simulink model "testerdolimiterow"  (R2022b)
settings: Solver=VariableStepAuto  StartTime=0.0  StopTime=10  RelTol=1e-3
values from neighbouring files (symbols this model uses):
  IPR = 0.99    [dane.m]    (also in tester23.m; wykresownik33.m; wykresownik35.m; wykresownik36.m)
  Ng_safe = 1.25    [dane.m]    (also in tester23.m; wykresownik33.m; wykresownik35.m; wykresownik36.m)
  No_perf = 1    [dane.m]    (also in tester23.m; wykresownik33.m; wykresownik35.m; wykresownik36.m)
  No_safe = 1.16    [dane.m]    (also in tester23.m; wykresownik33.m; wykresownik35.m; wykresownik36.m)
  Np = linspace(0.5,2,101)    [dane.m]    (also in tester23.m; untitled.m = 2303; wykresownik33.m; wykresownik35.m)
  Np_safe = 1.25    [dane.m]    (also in tester23.m; wykresownik33.m; wykresownik35.m; wykresownik36.m)
  P3tDIVP2t_perf = 1.0101    [dane.m]    (also in tester23.m = 1; wykresownik33.m = 1; wykresownik35.m = 1; wykresownik36.m = 1)
  Q = 1./Np    [dane.m]    (also in tester23.m; wykresownik33.m; wykresownik35.m; wykresownik36.m)
  Q_safe = 1.15    [dane.m]    (also in tester23.m; wykresownik33.m; wykresownik35.m; wykresownik36.m)
  T45_perf = 1    [dane.m]    (also in tester23.m; wykresownik33.m; wykresownik35.m; wykresownik36.m)
  T45_safe = 1.3    [dane.m]    (also in tester23.m; wykresownik33.m; wykresownik35.m; wykresownik36.m)
settings Model: Creator=48519  LastModifiedBy=48519
settings ModelReferenceCC: EnableRefExpFcnMdlSchedulingChecks=on

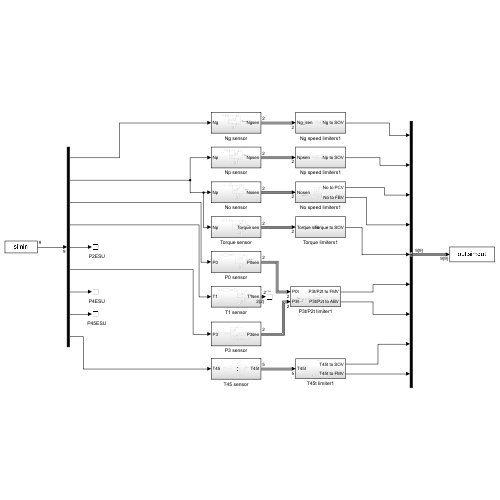
[thumbnail: Simulink's stored preview of the top-level diagram]
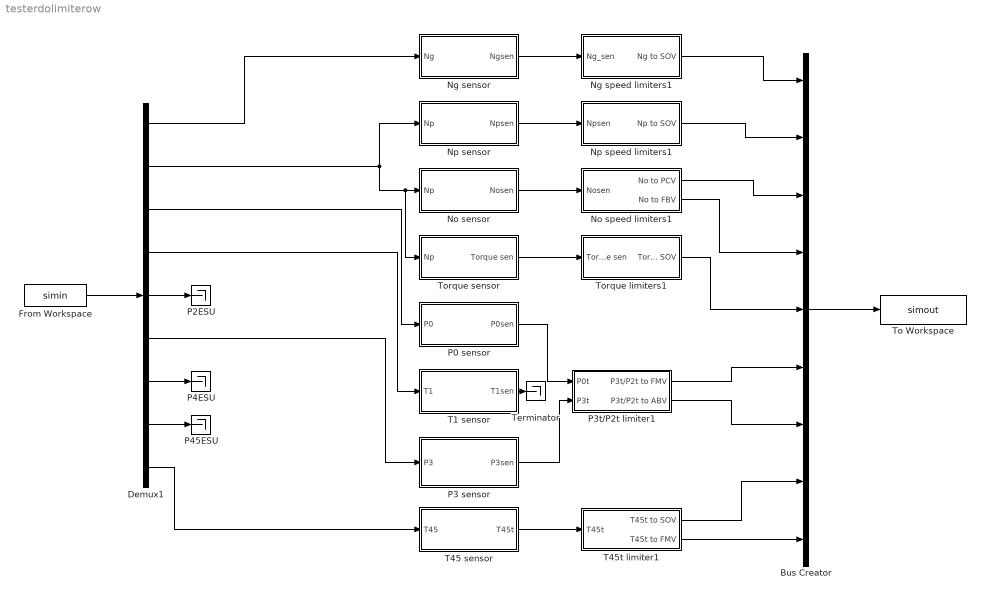
== system testerdolimiterow ==
  Bus Creator : BusCreator  Inputs=9
  Demux1 : Demux  Outputs=9
  From Workspace : FromWorkspace  VariableName=simin
  Ng sensor : Subsystem
  Ng speed limiters1 : Subsystem
  No sensor : Subsystem
  No speed limiters1 : Subsystem
  Np sensor : Subsystem
  Np speed limiters1 : Subsystem
  P0 sensor : Subsystem
  P2ESU : Terminator
  P3 sensor : Subsystem
  P3t/P2t limiter1 : Subsystem
  P45ESU : Terminator
  P4ESU : Terminator
  T1 sensor : Subsystem
  T45 sensor : Subsystem
  T45t limiter1 : Subsystem
  Terminator : Terminator
  To Workspace : ToWorkspace  VariableName=simout  SaveFormat=Timeseries  SampleTime=-1
  Torque limiters1 : Subsystem
  Torque sensor : Subsystem
  wires:
  Torque sensor/1(Torque sen) -> Torque limiters1/1(Torque sen)
  Ng sensor/1(Ngsen) -> Ng speed limiters1/1(Ng_sen)
  Demux1/2 -> Np sensor/1(Np), Torque sensor/1(Np), No sensor/1(Np)
  Demux1/1 -> Ng sensor/1(Ng)
  P3 sensor/1(P3sen) -> P3t/P2t limiter1/2(P3t)
  No sensor/1(Nosen) -> No speed limiters1/1(Nosen)
  P0 sensor/1(P0sen) -> P3t/P2t limiter1/1(P0t)
  From Workspace/1 -> Demux1/1
  Demux1/8 -> P45ESU/1
  Demux1/3 -> P0 sensor/1(P0)
  Demux1/6 -> P3 sensor/1(P3)
  Demux1/7 -> P4ESU/1
  Demux1/4 -> T1 sensor/1(T1)
  Demux1/5 -> P2ESU/1
  Demux1/9 -> T45 sensor/1(T45)
  Np sensor/1(Npsen) -> Np speed limiters1/1(Npsen)
  T45 sensor/1(T45t) -> T45t limiter1/1(T45t)
  T1 sensor/1(T1sen) -> Terminator/1
  P3t/P2t limiter1/2(P3t/P2t to ABV) -> Bus Creator/7
  Ng speed limiters1/1(Ng to SOV) -> Bus Creator/1
  T45t limiter1/1(T45t to SOV) -> Bus Creator/8
  Np speed limiters1/1(Np to SOV) -> Bus Creator/2
  No speed limiters1/1(No to PCV) -> Bus Creator/3
  Bus Creator/1 -> To Workspace/1
  No speed limiters1/2(No to FBV) -> Bus Creator/4
  P3t/P2t limiter1/1(P3t/P2t to FMV) -> Bus Creator/6
  T45t limiter1/2(T45t to FMV) -> Bus Creator/9
  Torque limiters1/1(Torque to SOV) -> Bus Creator/5

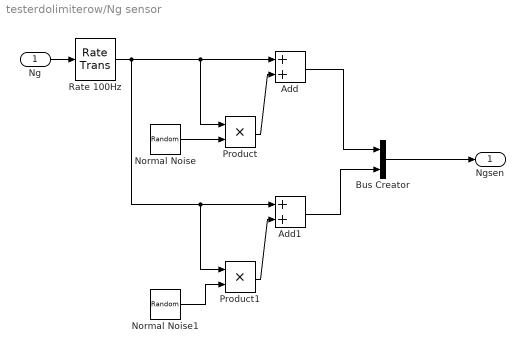
== system testerdolimiterow/Ng sensor ==
  Ng : Inport
  Add : Sum
  Add1 : Sum
  Bus Creator : BusCreator  Inputs=2
  Normal Noise : RandomNumber  Variance=((0.017)^2)*pi/2  Seed=10  SampleTime=0.01
  Normal Noise1 : RandomNumber  Variance=((0.017)^2)*pi/2  Seed=11  SampleTime=0.01
  Product : Product
  Product1 : Product
  Rate 100Hz : RateTransition  OutPortSampleTimeMultiple=2  OutPortSampleTime=0.01
  Ngsen : Outport
  wires:
  Product/1 -> Add/2
  Product1/1 -> Add1/2
  Normal Noise1/1 -> Product1/2
  Rate 100Hz/1 -> Add/1, Product/1, Add1/1, Product1/1
  Ng/1 -> Rate 100Hz/1
  Add1/1 -> Bus Creator/2
  Add/1 -> Bus Creator/1
  Bus Creator/1 -> Ngsen/1
  Normal Noise/1 -> Product/2

== system testerdolimiterow/Ng speed limiters1 ==
  Ng_sen : Inport
  Add : Sum
  Constant : Constant  Value=-1
  Constant1 : Constant
  Demux : Demux  Outputs=2
  Gain : Gain  Gain=0.5
  Safe switch : Subsystem
  Switch : Switch  Criteria=u2 > Threshold  Threshold=Ng_safe  SaturateOnIntegerOverflow=off  InputSameDT=off
  Ng to SOV : Outport
  wires:
  Constant/1 -> Switch/3
  Constant1/1 -> Switch/1
  Ng_sen/1 -> Demux/1
  Demux/1 -> Add/1
  Demux/2 -> Add/2
  Gain/1 -> Switch/2
  Add/1 -> Gain/1
  Switch/1 -> Safe switch/1(In1)
  Safe switch/1(Out1) -> Ng to SOV/1

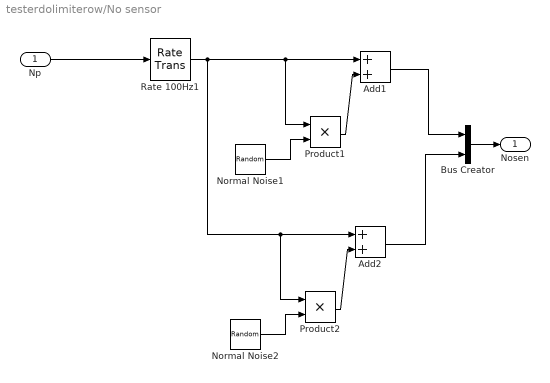
== system testerdolimiterow/No sensor ==
  Np : Inport
  Add1 : Sum
  Add2 : Sum
  Bus Creator : BusCreator  Inputs=2
  Normal Noise1 : RandomNumber  Variance=((0.017)^2)*pi/2  Seed=16  SampleTime=0.01
  Normal Noise2 : RandomNumber  Variance=((0.017)^2)*pi/2  Seed=18  SampleTime=0.01
  Product1 : Product
  Product2 : Product
  Rate 100Hz1 : RateTransition  OutPortSampleTimeMultiple=2  OutPortSampleTime=0.01
  Nosen : Outport
  wires:
  Np/1 -> Rate 100Hz1/1
  Normal Noise2/1 -> Product2/2
  Rate 100Hz1/1 -> Add2/1, Product2/1, Add1/1, Product1/1
  Add2/1 -> Bus Creator/2
  Add1/1 -> Bus Creator/1
  Bus Creator/1 -> Nosen/1
  Normal Noise1/1 -> Product1/2
  Product1/1 -> Add1/2
  Product2/1 -> Add2/2

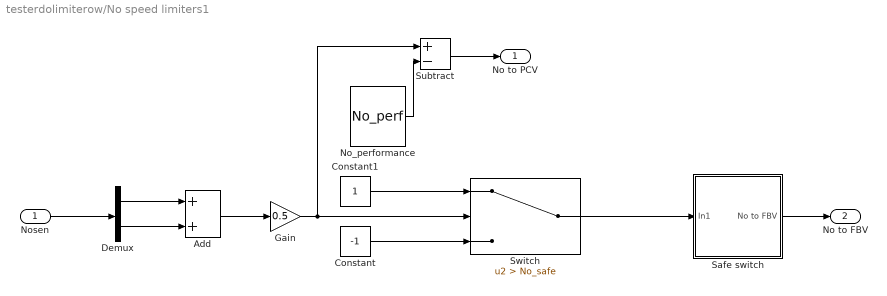
== system testerdolimiterow/No speed limiters1 ==
  Nosen : Inport
  Add : Sum
  Constant : Constant  Value=-1
  Constant1 : Constant
  Demux : Demux  Outputs=2
  Gain : Gain  Gain=0.5
  No_performance : Constant  Value=No_perf
  Safe switch : Subsystem
  Subtract : Sum  Inputs=+-
  Switch : Switch  Criteria=u2 > Threshold  Threshold=No_safe  SaturateOnIntegerOverflow=off  InputSameDT=off
  No to PCV : Outport
  No to FBV : Outport  Port=2
  wires:
  Add/1 -> Gain/1
  Nosen/1 -> Demux/1
  Demux/1 -> Add/1
  Demux/2 -> Add/2
  Constant/1 -> Switch/3
  Constant1/1 -> Switch/1
  Gain/1 -> Subtract/1, Switch/2
  No_performance/1 -> Subtract/2
  Subtract/1 -> No to PCV/1
  Switch/1 -> Safe switch/1(In1)
  Safe switch/1(No to FBV) -> No to FBV/1

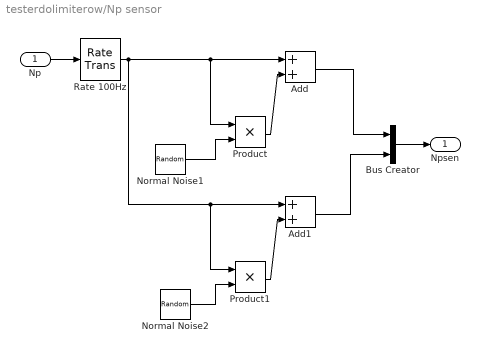
== system testerdolimiterow/Np sensor ==
  Np : Inport
  Add : Sum
  Add1 : Sum
  Bus Creator : BusCreator  Inputs=2
  Normal Noise1 : RandomNumber  Variance=((0.017)^2)*pi/2  Seed=13  SampleTime=0.01
  Normal Noise2 : RandomNumber  Variance=((0.017)^2)*pi/2  Seed=14  SampleTime=0.01
  Product : Product
  Product1 : Product
  Rate 100Hz : RateTransition  OutPortSampleTimeMultiple=2  OutPortSampleTime=0.01
  Npsen : Outport
  wires:
  Normal Noise1/1 -> Product/2
  Product/1 -> Add/2
  Np/1 -> Rate 100Hz/1
  Normal Noise2/1 -> Product1/2
  Product1/1 -> Add1/2
  Rate 100Hz/1 -> Add/1, Product/1, Add1/1, Product1/1
  Add1/1 -> Bus Creator/2
  Add/1 -> Bus Creator/1
  Bus Creator/1 -> Npsen/1

== system testerdolimiterow/Np speed limiters1 ==
  Npsen : Inport
  Add : Sum
  Constant : Constant  Value=-1
  Constant1 : Constant
  Demux : Demux  Outputs=2
  Gain : Gain  Gain=0.5
  Safe switch : Subsystem
  Switch : Switch  Criteria=u2 > Threshold  Threshold=Np_safe  SaturateOnIntegerOverflow=off  InputSameDT=off
  Np to SOV : Outport
  wires:
  Switch/1 -> Safe switch/1(In1)
  Constant1/1 -> Switch/1
  Constant/1 -> Switch/3
  Gain/1 -> Switch/2
  Demux/2 -> Add/2
  Npsen/1 -> Demux/1
  Add/1 -> Gain/1
  Demux/1 -> Add/1
  Safe switch/1(Np to SOV) -> Np to SOV/1

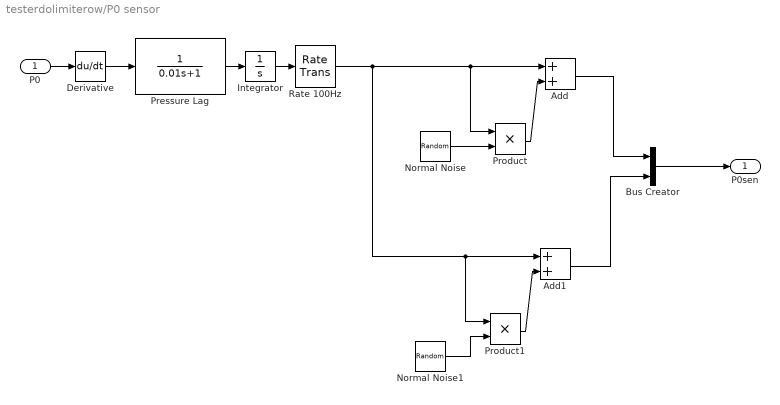
== system testerdolimiterow/P0 sensor ==
  P0 : Inport
  Add : Sum
  Add1 : Sum
  Bus Creator : BusCreator  Inputs=2
  Derivative : Derivative
  Integrator : Integrator  InitialCondition=1
  Normal Noise : RandomNumber  Variance=((0.005)^2)*pi/2  Seed=31  SampleTime=0.01
  Normal Noise1 : RandomNumber  Variance=((0.005)^2)*pi/2  Seed=33  SampleTime=0.01
  Pressure Lag : TransferFcn  Denominator=[0.01 1]
  Product : Product
  Product1 : Product
  Rate 100Hz : RateTransition  OutPortSampleTimeMultiple=2  OutPortSampleTime=0.01
  P0sen : Outport
  wires:
  P0/1 -> Derivative/1
  Normal Noise1/1 -> Product1/2
  Normal Noise/1 -> Product/2
  Add1/1 -> Bus Creator/2
  Pressure Lag/1 -> Integrator/1
  Bus Creator/1 -> P0sen/1
  Product1/1 -> Add1/2
  Product/1 -> Add/2
  Rate 100Hz/1 -> Add1/1, Product1/1, Add/1, Product/1
  Add/1 -> Bus Creator/1
  Derivative/1 -> Pressure Lag/1
  Integrator/1 -> Rate 100Hz/1

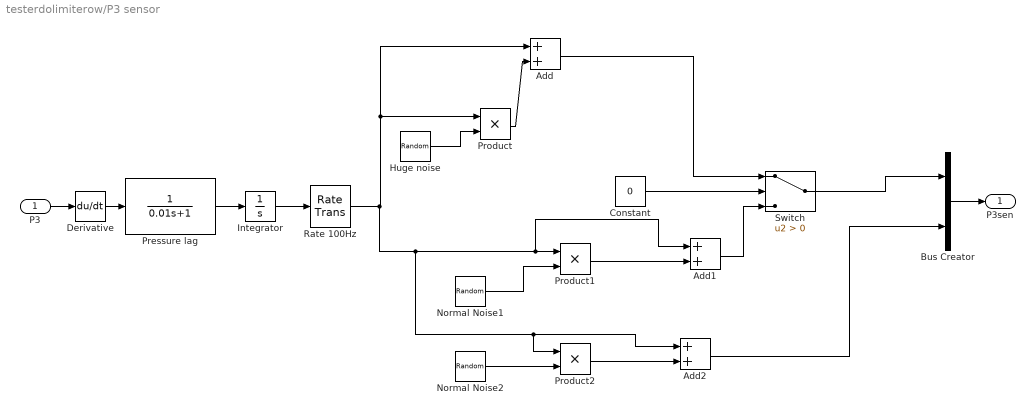
== system testerdolimiterow/P3 sensor ==
  P3 : Inport
  Add : Sum
  Add1 : Sum
  Add2 : Sum
  Bus Creator : BusCreator  Inputs=2
  Constant : Constant  Value=0
  Derivative : Derivative
  Huge noise : RandomNumber  Variance=((0.03)^2)*pi/2  Seed=1  SampleTime=0.01
  Integrator : Integrator  InitialCondition=1
  Normal Noise1 : RandomNumber  Variance=((0.005)^2)*pi/2  Seed=2  SampleTime=0.01
  Normal Noise2 : RandomNumber  Variance=((0.005)^2)*pi/2  Seed=4  SampleTime=0.01
  Pressure lag : TransferFcn  Numerator=[1 ]  Denominator=[0.01 1]
  Product : Product
  Product1 : Product
  Product2 : Product
  Rate 100Hz : RateTransition  OutPortSampleTimeMultiple=2  OutPortSampleTime=0.01
  Switch : Switch  Criteria=u2 > Threshold  SaturateOnIntegerOverflow=off  InputSameDT=off
  P3sen : Outport
  wires:
  Bus Creator/1 -> P3sen/1
  P3/1 -> Derivative/1
  Normal Noise2/1 -> Product2/2
  Add/1 -> Switch/1
  Huge noise/1 -> Product/2
  Add1/1 -> Switch/3
  Product/1 -> Add/2
  Product2/1 -> Add2/2
  Rate 100Hz/1 -> Add2/1, Product2/1, Add1/1, Product1/1, Product/1, Add/1
  Add2/1 -> Bus Creator/2
  Normal Noise1/1 -> Product1/2
  Switch/1 -> Bus Creator/1
  Pressure lag/1 -> Integrator/1
  Constant/1 -> Switch/2
  Product1/1 -> Add1/2
  Derivative/1 -> Pressure lag/1
  Integrator/1 -> Rate 100Hz/1

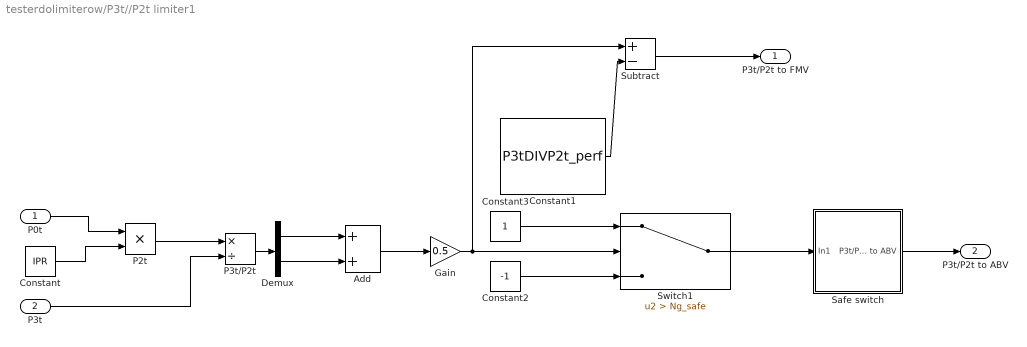
== system testerdolimiterow/P3t//P2t limiter1 ==
  P0t : Inport
  P3t : Inport  Port=2
  Add : Sum
  Constant : Constant  Value=IPR
  Constant1 : Constant  Value=P3tDIVP2t_perf
  Constant2 : Constant  Value=-1
  Constant3 : Constant
  Demux : Demux  Outputs=2
  Gain : Gain  Gain=0.5
  P2t : Product
  P3t/P2t : Product  Inputs=*/
  Safe switch : Subsystem
  Subtract : Sum  Inputs=+-
  Switch1 : Switch  Criteria=u2 > Threshold  Threshold=Ng_safe  SaturateOnIntegerOverflow=off  InputSameDT=off
  P3t/P2t to FMV : Outport
  P3t/P2t to ABV : Outport  Port=2
  wires:
  Subtract/1 -> P3t/P2t to FMV/1
  P3t/1 -> P3t/P2t/2
  P0t/1 -> P2t/1
  P2t/1 -> P3t/P2t/1
  Constant/1 -> P2t/2
  Constant1/1 -> Subtract/2
  Constant2/1 -> Switch1/3
  Switch1/1 -> Safe switch/1(In1)
  Constant3/1 -> Switch1/1
  Demux/2 -> Add/2
  Demux/1 -> Add/1
  Add/1 -> Gain/1
  P3t/P2t/1 -> Demux/1
  Gain/1 -> Subtract/1, Switch1/2
  Safe switch/1(P3t/P2t to ABV) -> P3t/P2t to ABV/1

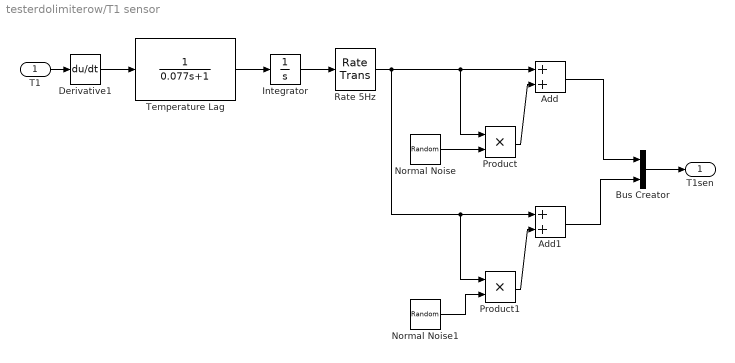
== system testerdolimiterow/T1 sensor ==
  T1 : Inport
  Add : Sum
  Add1 : Sum
  Bus Creator : BusCreator  Inputs=2
  Derivative1 : Derivative
  Integrator : Integrator  InitialCondition=1
  Normal Noise : RandomNumber  Variance=((0.01)^2)*pi/2  Seed=41  SampleTime=0.2
  Normal Noise1 : RandomNumber  Variance=((0.01)^2)*pi/2  Seed=42  SampleTime=0.2
  Product : Product
  Product1 : Product
  Rate 5Hz : RateTransition  OutPortSampleTimeMultiple=2  OutPortSampleTime=0.2
  Temperature Lag : TransferFcn  Denominator=[0.077 1]
  T1sen : Outport
  wires:
  T1/1 -> Derivative1/1
  Temperature Lag/1 -> Integrator/1
  Derivative1/1 -> Temperature Lag/1
  Normal Noise1/1 -> Product1/2
  Normal Noise/1 -> Product/2
  Add1/1 -> Bus Creator/2
  Bus Creator/1 -> T1sen/1
  Rate 5Hz/1 -> Add/1, Product/1, Add1/1, Product1/1
  Add/1 -> Bus Creator/1
  Product1/1 -> Add1/2
  Product/1 -> Add/2
  Integrator/1 -> Rate 5Hz/1

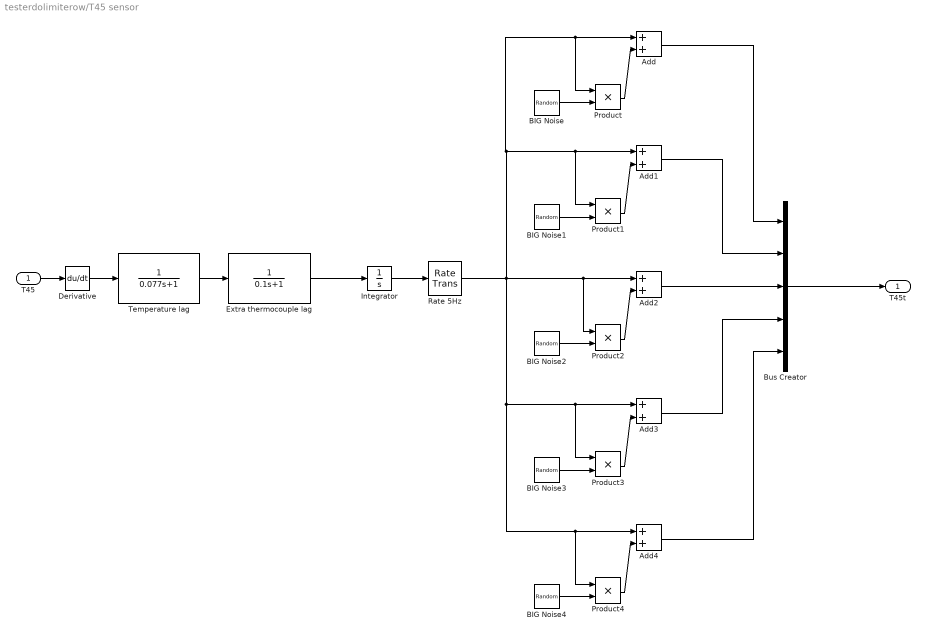
== system testerdolimiterow/T45 sensor ==
  T45 : Inport
  Add{,1..4} (5 alike) : Sum
  BIG Noise : RandomNumber  Variance=((0.015)^2)*pi/2  Seed=51  SampleTime=0.2
  BIG Noise1 : RandomNumber  Variance=((0.015)^2)*pi/2  Seed=53  SampleTime=0.2
  BIG Noise2 : RandomNumber  Variance=((0.015)^2)*pi/2  Seed=55  SampleTime=0.2
  BIG Noise3 : RandomNumber  Variance=((0.015)^2)*pi/2  Seed=57  SampleTime=0.2
  BIG Noise4 : RandomNumber  Variance=((0.015)^2)*pi/2  Seed=59  SampleTime=0.2
  Bus Creator : BusCreator  Inputs=5
  Derivative : Derivative
  Extra thermocouple lag : TransferFcn  Denominator=[0.1 1]
  Integrator : Integrator  InitialCondition=1
  Product{,1..4} (5 alike) : Product
  Rate 5Hz : RateTransition  OutPortSampleTime=0.2
  Temperature lag : TransferFcn  Denominator=[0.077 1]
  T45t : Outport
  wires:
  T45/1 -> Derivative/1
  Extra thermocouple lag/1 -> Integrator/1
  Temperature lag/1 -> Extra thermocouple lag/1
  BIG Noise/1 -> Product/2
  Product/1 -> Add/2
  Product1/1 -> Add1/2
  BIG Noise1/1 -> Product1/2
  Product2/1 -> Add2/2
  BIG Noise2/1 -> Product2/2
  Product3/1 -> Add3/2
  BIG Noise3/1 -> Product3/2
  Product4/1 -> Add4/2
  Rate 5Hz/1 -> Add/1, Product/1, Add1/1, Product1/1, Product2/1, Add2/1, Add3/1, Product3/1, Add4/1, Product4/1
  BIG Noise4/1 -> Product4/2
  Bus Creator/1 -> T45t/1
  Add2/1 -> Bus Creator/3
  Add3/1 -> Bus Creator/4
  Add4/1 -> Bus Creator/5
  Add1/1 -> Bus Creator/2
  Add/1 -> Bus Creator/1
  Integrator/1 -> Rate 5Hz/1
  Derivative/1 -> Temperature lag/1

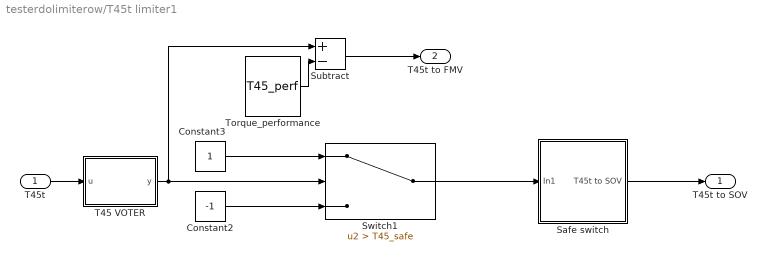
== system testerdolimiterow/T45t limiter1 ==
  T45t : Inport
  Constant2 : Constant  Value=-1
  Constant3 : Constant
  Safe switch : Subsystem
  Subtract : Sum  Inputs=+-
  Switch1 : Switch  Criteria=u2 > Threshold  Threshold=T45_safe  SaturateOnIntegerOverflow=off  InputSameDT=off
  T45 VOTER : MATLAB Function  TreatAsAtomicUnit=on
  Torque_performance : Constant  Value=T45_perf
  T45t to SOV : Outport
  T45t to FMV : Outport  Port=2
  wires:
  Subtract/1 -> T45t to FMV/1
  ? -> ?
  Switch1/1 -> Safe switch/1(In1)
  Constant2/1 -> Switch1/3
  Constant3/1 -> Switch1/1
  Torque_performance/1 -> Subtract/2
  T45 VOTER/1(y) -> Subtract/1, Switch1/2
  T45t/1 -> T45 VOTER/1(u)
  Safe switch/1(T45t to SOV) -> T45t to SOV/1

== system testerdolimiterow/Torque limiters1 ==
  Torque sen : Inport
  Add : Sum
  Constant : Constant  Value=-1
  Constant1 : Constant
  Demux : Demux  Outputs=2
  Gain : Gain  Gain=0.5
  Safe switch : Subsystem
  Switch : Switch  Criteria=u2 > Threshold  Threshold=Q_safe  SaturateOnIntegerOverflow=off  InputSameDT=off
  Torque to SOV : Outport
  wires:
  Gain/1 -> Switch/2
  Constant1/1 -> Switch/1
  Torque sen/1 -> Demux/1
  Constant/1 -> Switch/3
  Demux/2 -> Add/2
  Add/1 -> Gain/1
  Demux/1 -> Add/1
  Switch/1 -> Safe switch/1(In1)
  Safe switch/1(Torque to SOV) -> Torque to SOV/1

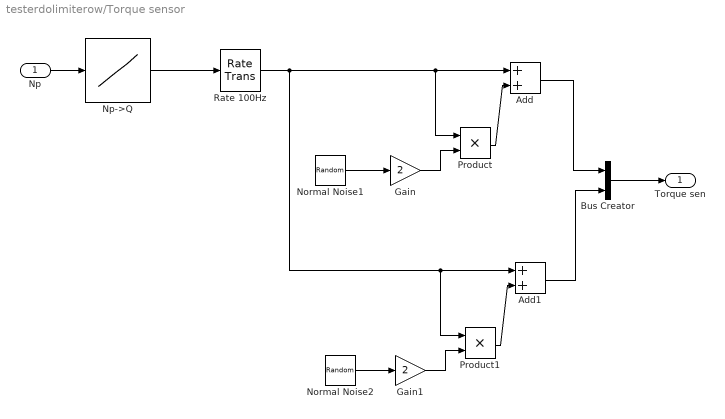
== system testerdolimiterow/Torque sensor ==
  Np : Inport
  Add : Sum
  Add1 : Sum
  Bus Creator : BusCreator  Inputs=2
  Gain : Gain  Gain=2
  Gain1 : Gain  Gain=2
  Normal Noise1 : RandomNumber  Variance=((0.017)^2)*pi/2  Seed=21  SampleTime=0.01
  Normal Noise2 : RandomNumber  Variance=((0.017)^2)*pi/2  Seed=23  SampleTime=0.01
  Np->Q : Lookup_n-D  NumberOfTableDimensions=1  BreakpointsForDimension1=Np  Table=Q  InternalRulePriority=Speed  RndMeth=Simplest
  Product : Product
  Product1 : Product
  Rate 100Hz : RateTransition  OutPortSampleTimeMultiple=2  OutPortSampleTime=0.01
  Torque sen : Outport
  wires:
  Normal Noise1/1 -> Gain/1
  Product/1 -> Add/2
  Gain/1 -> Product/2
  Normal Noise2/1 -> Gain1/1
  Product1/1 -> Add1/2
  Gain1/1 -> Product1/2
  Rate 100Hz/1 -> Add1/1, Product1/1, Add/1, Product/1
  Add1/1 -> Bus Creator/2
  Np/1 -> Np->Q/1
  Add/1 -> Bus Creator/1
  Bus Creator/1 -> Torque sen/1
  Np->Q/1 -> Rate 100Hz/1

== system testerdolimiterow/Ng speed limiters1/Safe switch ==
  In1 : Inport
  Add1 : Sum
  Delay : Delay  DelayLength=1
  OFF : Constant  Value=0
  ON : Constant
  Switch1 : Switch  Criteria=u2 > Threshold  Threshold=10  SaturateOnIntegerOverflow=off  InputSameDT=off
  min 0 : Saturate  UpperLimit=100  LowerLimit=0
  Out1 : Outport
  wires:
  ON/1 -> Switch1/1
  Delay/1 -> Add1/2
  Add1/1 -> min 0/1
  Switch1/1 -> Out1/1
  min 0/1 -> Switch1/2, Delay/1
  OFF/1 -> Switch1/3
  In1/1 -> Add1/1

== system testerdolimiterow/No speed limiters1/Safe switch ==
  In1 : Inport
  Add1 : Sum
  Delay : Delay  DelayLength=1
  OFF : Constant  Value=0
  ON : Constant
  Switch1 : Switch  Criteria=u2 > Threshold  Threshold=10  SaturateOnIntegerOverflow=off  InputSameDT=off
  min 0 : Saturate  UpperLimit=100  LowerLimit=0
  No to FBV : Outport
  wires:
  ON/1 -> Switch1/1
  Delay/1 -> Add1/2
  Add1/1 -> min 0/1
  Switch1/1 -> No to FBV/1
  min 0/1 -> Switch1/2, Delay/1
  OFF/1 -> Switch1/3
  In1/1 -> Add1/1

== system testerdolimiterow/Np speed limiters1/Safe switch ==
  In1 : Inport
  Add1 : Sum
  Delay : Delay  DelayLength=1
  OFF : Constant  Value=0
  ON : Constant
  Switch1 : Switch  Criteria=u2 > Threshold  Threshold=10  SaturateOnIntegerOverflow=off  InputSameDT=off
  min 0 : Saturate  UpperLimit=100  LowerLimit=0
  Np to SOV : Outport
  wires:
  ON/1 -> Switch1/1
  Delay/1 -> Add1/2
  Add1/1 -> min 0/1
  Switch1/1 -> Np to SOV/1
  min 0/1 -> Switch1/2, Delay/1
  OFF/1 -> Switch1/3
  In1/1 -> Add1/1

== system testerdolimiterow/P3t//P2t limiter1/Safe switch ==
  In1 : Inport
  Add1 : Sum
  Delay : Delay  DelayLength=1
  OFF : Constant  Value=0
  ON : Constant
  Switch1 : Switch  Criteria=u2 > Threshold  Threshold=10  SaturateOnIntegerOverflow=off  InputSameDT=off
  min 0 : Saturate  UpperLimit=100  LowerLimit=0
  P3t/P2t to ABV : Outport
  wires:
  ON/1 -> Switch1/1
  Delay/1 -> Add1/2
  Add1/1 -> min 0/1
  Switch1/1 -> P3t/P2t to ABV/1
  min 0/1 -> Switch1/2, Delay/1
  OFF/1 -> Switch1/3
  In1/1 -> Add1/1

== system testerdolimiterow/T45t limiter1/Safe switch ==
  In1 : Inport
  Add1 : Sum
  Delay : Delay  DelayLength=1
  OFF : Constant  Value=0
  ON : Constant
  Switch1 : Switch  Criteria=u2 > Threshold  Threshold=10  SaturateOnIntegerOverflow=off  InputSameDT=off
  min 0 : Saturate  UpperLimit=100  LowerLimit=0
  T45t to SOV : Outport
  wires:
  ON/1 -> Switch1/1
  Delay/1 -> Add1/2
  Add1/1 -> min 0/1
  Switch1/1 -> T45t to SOV/1
  min 0/1 -> Switch1/2, Delay/1
  OFF/1 -> Switch1/3
  In1/1 -> Add1/1

== system testerdolimiterow/Torque limiters1/Safe switch ==
  In1 : Inport
  Add1 : Sum
  Delay : Delay  DelayLength=1
  OFF : Constant  Value=0
  ON : Constant
  Switch1 : Switch  Criteria=u2 > Threshold  Threshold=10  SaturateOnIntegerOverflow=off  InputSameDT=off
  min 0 : Saturate  UpperLimit=100  LowerLimit=0
  Torque to SOV : Outport
  wires:
  ON/1 -> Switch1/1
  Delay/1 -> Add1/2
  Add1/1 -> min 0/1
  Switch1/1 -> Torque to SOV/1
  min 0/1 -> Switch1/2, Delay/1
  OFF/1 -> Switch1/3
  In1/1 -> Add1/1

== matlab function testerdolimiterow/T45t limiter1/T45 VOTER ==
  data: u input; y output
function y = fcn(u)
u=sort(u);
y = (u(2)+u(3)+u(4))/3;
